simulink model "raibert_hopper_2d"  (R2014b)
settings: Solver=FixedStepDiscrete  StartTime=0.0  StopTime=inf  FixedStep=sample_time  RelTol=1e-3
undefined symbols (not defined in the file): boom_mount_angle, boom_pelvis_offset_angle, contact_threshold, control_start_time, d_y_boom_com_offset, desired_torso_angle, dt_thrust, dx_avg_desired, dx_avg_samples, dx_desired_step, extra_leg_damping, F_thrust, fcut_contact, g, h_boom, HIP_MTR_MAX_CONT_TORQUE, initial_dt, k_placement, k_sea, kd_flight, kd_lateral, kd_leg_angle, kd_leg_length_secondary, kd_torso, kd_virtual, kp_flight_max, kp_flight_min, kp_lateral, kp_leg_angle, kp_leg_length_secondary, kp_torso, kp_virtual, l0_virtual, l_boom_projected, l_max, l_min, l_retract, l_seg, l_yaw_center_to_pelvis, lambda1, lambda2, lateral_offset, lateral_target_angle_left, lateral_target_angle_right, leg_length_secondary, loaded_threshold, m_leg_motor, m_total_real, max_leg_angle, max_torque_lateral, max_torque_sagittal, maximum_lateral_angle, min_leg_angle, minimum_lateral_angle, sample_time, t_flight, x_limit
libraries: simulink x7
(part 2 of 2)

== matlab function raibert_hopper_2d/Control/Behavior Control/Torque Distribution Left/Motor Torque Saturation Optimization ==
  data: x1s input; t1 output; x2s input; lambda1 parameter; lambda2 parameter; max_torque_sagittal parameter; t2 output
% Optimal leg motor torque distribution
function [t1, t2] = distribute_torque(x1s, x2s, lambda1, lambda2, max_torque_sagittal)

s = max_torque_sagittal;

% possible solutions
x1 = [                                                      x1s;
                                                            0;
                                                            s;
                                                            0;
                                                           -s;
  (lambda2*s + lambda1*x1s - lambda2*x2s)/(lambda1 + lambda2);
  (lambda1*x1s - lambda2*s + lambda2*x2s)/(lambda1 + lambda2);
  (lambda2*s + lambda1*x1s + lambda2*x2s)/(lambda1 + lambda2);
 -(lambda2*s - lambda1*x1s + lambda2*x2s)/(lambda1 + lambda2)];
 
x2 = [                                                      x2s;
                                                            s;
                                                            0;
                                                           -s;
                                                            0;
  (lambda1*s - lambda1*x1s + lambda2*x2s)/(lambda1 + lambda2);
  (lambda1*s + lambda1*x1s + lambda2*x2s)/(lambda1 + lambda2);
  (lambda1*x1s - lambda1*s + lambda2*x2s)/(lambda1 + lambda2);
 -(lambda1*s + lambda1*x1s - lambda2*x2s)/(lambda1 + lambda2)];

% test constraints
c1 = s - x1 - x2 >= 0;
c2 = s + x1 + x2 >= 0;
c3 = s - x1 + x2 >= 0;
c4 = s + x1 - x2 >= 0;
constraints = c1 & c2 & c3 & c4;

% objective function to maximize
f = -lambda1*(x1-x1s).^2-lambda2*(x2-x2s).^2;
satisfied = find(constraints);
[~,I] = max(f(satisfied));

t1 = x1(satisfied(I));
t2 = x2(satisfied(I));
